simulink model "Speed_from_Force_Slider"  (R2021a)
settings: Solver=VariableStepAuto  StartTime=0.0  StopTime=1000  RelTol=1e-3
settings Model: Creator=Yogesh  LastModifiedBy=Yogesh

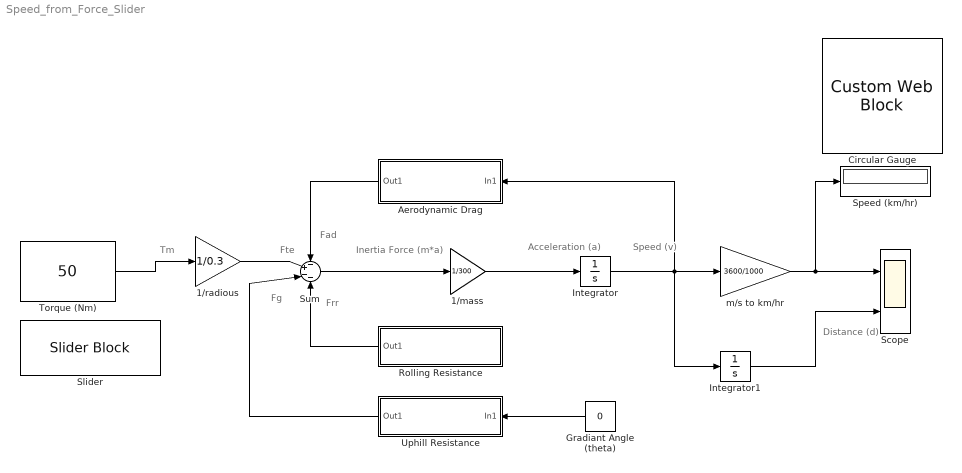
== system Speed_from_Force_Slider ==
  note: Fte
  note: Fad
  note: Fg
  note: Frr
  note: Inertia Force
      | (m*a)
  note: Acceleration
      | (a)
  note: Speed
      | (v)
  note: Distance
      | (d)
  note: Tm
  1/mass : Gain  Gain=1/300
  1/radious : Gain  Gain=1/0.3
  Aerodynamic Drag : Subsystem
  Circular Gauge : CustomWebBlock  LabelPosition=Hide  ShowInitialText=on  Configuration="{\"components\":[{\"name\":\"CircularScaleComponent\",\"settings\":{\"bounds\":{\"max\":100,\"min\":0,\"tickInterval\":\"auto\"},\"direction\":\"cw\",\"flipLimits\":0,\"innerRadius\":0.75,\"internalTickHeightScaleFactor\":1,\"labelColor\":[255,255,200],\"labelFont\":{\"font\":\"Arial\",\"fontSize\":12},\"labelTransparency\":1,\"minorTickHeightScaleFactor\":0.2,\"needleImage\":{\"size\":[200,50],\"src\":\"data:image\\/svg+xml;base64,PD94bWwgdmVyc2lvbj0iMS4wIiBlbmNvZGluZz0idXRmLTgiPz4KPCEtLSBHZW5lcmF0b3I6IEFkb2JlIElsbHVzdHJhdG9yIDI0LjEuMiwgU1ZHIEV4cG9ydCBQbHVnLUluIC4gU1ZHIFZlcnNpb246IDYuMDAgQnVpbGQgMCkgIC0tPgo8c3ZnIHZlcnNpb249IjEuMSIgaWQ9IkxheWVyXzEiIHhtbG5zPSJodHRwOi8vd3d3LnczLm9yZy8yMDAwL3N2ZyIgeG1sbnM6eGxpbms9Imh0dHA6Ly93d3cudzMub3JnLzE5OTkveGxpbmsiIHg9IjBweCIgeT0iMHB4IgoJIHZpZXdCb3g9IjAgMCAyMDAgNTAiIHN0eWxlPSJlbmFibGUtYmFja2dyb3VuZDpuZXcgMCAwIDIwMCA1MDsiIHhtbDpzcGFjZT0icHJlc2VydmUiPgo8c3R5bGUgdHlwZT0idGV4dC9jc3MiPgoJLnN0MHtmaWxsOiNFQzIxMjc7fQo8L3N0eWxlPgo8cGF0aCBjbGFzcz0ic3QwIiBkPSJNMTYyLjgsMTMuN0MxNjksNC40LDE4MS43LDEuOSwxOTEsOC4xczExLjgsMTguOSw1LjYsMjguMnMtMTguOSwxMS44LTI4LjIsNS42bDAsMAoJQzE1OS4xLDM1LjYsMTU2LjYsMjMsMTYyLjgsMTMuN0wxNjIuOCwxMy43eiBNMTY1LjgsMTUuOGMtNS4xLDcuNi0zLjEsMTcuOSw0LjYsMjNjNy42LDUuMSwxNy45LDMuMSwyMy00LjYKCWM1LjEtNy42LDMuMS0xNy45LTQuNi0yM2wwLDBDMTgxLjIsNi4yLDE3MC45LDguMiwxNjUuOCwxNS44eiIvPgo8cGF0aCBjbGFzcz0ic3QwIiBkPSJNMC40LDI1Ljl2LTMuM2wxNTktMi41Yy0wLjcsMi42LTAuNyw1LjIsMCw3LjhMMC40LDI1Ljl6Ii8+CjxjaXJjbGUgY2xhc3M9InN0MCIgY3g9IjE3OS42IiBjeT0iMjQiIHI9IjAuNyIvPgo8L3N2Zz4K\"},\"needleOffset\":[0.18464878250906522,0],\"needleOrientation\":-45,\"needleRotation\":180,\"needleSize\":{\"height\":0.11741692305346914,\"width\":0.46108337545091255},\"outerRadius\":0.9,\"position\":[0.06486742424242424,0.05627705627705628,0.8917748917748918,0.8787878787878788],\"scaleAngle\":270,\"scaleAngleOffset\":135,\"scaleColors\":[],\"scaleColorsSize\":0.2,\"scalePosition\":[0,0,1,1],\"showLabels\":1,\"showMinorTicks\":1,\"showSpanLine\":1,\"showTicks\":1,\"tickColor\":[252,252,197],\"tickTransparency\":1,\"valueBarColor\":[0,114,189],\"valueBarPosition\":[0,0,1,1],\"valueBarSize\":0.2,\"valueBarTransparency\":1}},{\"name\":\"BackgroundImageComponent\",\"settings\":{\"image\":{\"size\":[500,500],\"src\":\"data:image\\/svg+xml;base64,PD94bWwgdmVyc2lvbj0iMS4wIiBlbmNvZGluZz0iVVRGLTgiIHN0YW5kYWxvbmU9Im5vIj8+CjxzdmcKICAgeG1sbnM6ZGM9Imh0dHA6Ly9wdXJsLm9yZy9kYy9lbGVtZW50cy8xLjEvIgogICB4bWxuczpjYz0iaHR0cDovL2NyZWF0aXZlY29tbW9ucy5vcmcvbnMjIgogICB4bWxuczpyZGY9Imh0dHA6Ly93d3cudzMub3JnLzE5OTkvMDIvMjItcmRmLXN5bnRheC1ucyMiCiAgIHhtbG5zOnN2Zz0iaHR0cDovL3d3dy53My5vcmcvMjAwMC9zdmciCiAgIHhtbG5zPSJodHRwOi8vd3d3LnczLm9yZy8yMDAwL3N2ZyIKICAgeG1sbnM6 ...(+9964 chars)\"},\"position\":[0,0,1,1],\"scaleMode\":\"0\"}},{\"name\":\"ForegroundImageComponent\",\"settings\":{\"image\":{\"size\":[0,0],\"src\":\"default\",\"srcOrientation\":[]},\"isForeground\":1,\"position\":[0,0,1,1],\"scaleMode\":\"0\"}}],\"settings\":{\"BindingType\":\"signal\",\"aspectRatio\":1.032258064516129,\"backgroundColor\":[0,0,0,\"1\"],\"backgroundOffset\":0.14,\"backgroundOpacity\":1,\"direction\":\"cw\",\"fixedAspectRatio\":\"on\",\"flipLimits\":0,\"orientation\":\"horizontal\",\"showBackgroundColor\":false,\"value\":0},\"type\":\"CircularGauge\"}"
  Gradiant Angle (theta) : Constant  Value=0
  Integrator : Integrator
  Integrator1 : Integrator
  Rolling Resistance : Subsystem
  Scope : Scope  NumInputPorts=2
  Slider : SliderBlock  LabelPosition=Bottom
  Speed (km/hr) : Display
  Sum : Sum  Inputs=-+--
  Torque (Nm) : Constant  Value=50
  Uphill Resistance : Subsystem
  m/s to km/hr : Gain  Gain=3600/1000
  wires:
  Sum/1 -> 1/mass/1
  1/radious/1 -> Sum/2
  1/mass/1 -> Integrator/1
  Integrator/1 -> Aerodynamic Drag/1(In1), m/s to km/hr/1, Integrator1/1
  Aerodynamic Drag/1(Out1) -> Sum/1
  Gradiant Angle (theta)/1 -> Uphill Resistance/1(In1)
  Uphill Resistance/1(Out1) -> Sum/3
  m/s to km/hr/1 -> Speed (km/hr)/1, Scope/1
  Rolling Resistance/1(Out1) -> Sum/4
  Integrator1/1 -> Scope/2
  Torque (Nm)/1 -> 1/radious/1

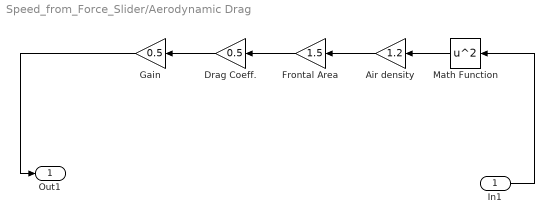
== system Speed_from_Force_Slider/Aerodynamic Drag ==
  In1 : Inport
  Air density : Gain  Gain=1.2
  Drag Coeff. : Gain  Gain=0.5
  Frontal Area : Gain  Gain=1.5
  Gain : Gain  Gain=0.5
  Math Function : Math  Operator=square  SaturateOnIntegerOverflow=on
  Out1 : Outport
  wires:
  Math Function/1 -> Air density/1
  Air density/1 -> Frontal Area/1
  Drag Coeff./1 -> Gain/1
  Frontal Area/1 -> Drag Coeff./1
  Gain/1 -> Out1/1
  In1/1 -> Math Function/1

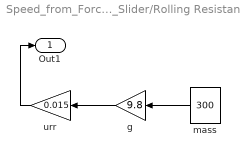
== system Speed_from_Force_Slider/Rolling Resistance ==
  g : Gain  Gain=9.8
  mass : Constant  Value=300
  urr : Gain  Gain=0.015
  Out1 : Outport
  wires:
  g/1 -> urr/1
  mass/1 -> g/1
  urr/1 -> Out1/1

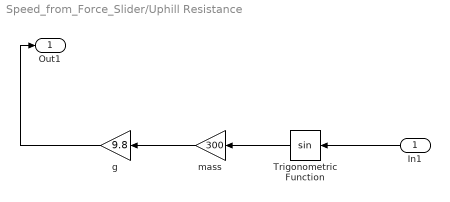
== system Speed_from_Force_Slider/Uphill Resistance ==
  In1 : Inport
  Trigonometric Function : Trigonometry
  g : Gain  Gain=9.8
  mass : Gain  Gain=300
  Out1 : Outport
  wires:
  In1/1 -> Trigonometric Function/1
  mass/1 -> g/1
  g/1 -> Out1/1
  Trigonometric Function/1 -> mass/1
